simulink library "rocket_isa_model_library"  (R2014a)
settings: Solver=ode45  StartTime=0.0  StopTime=10.0  RelTol=1e-3
settings Model: Creator=scorpii  LastModifiedBy=scorpii

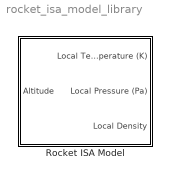
== system rocket_isa_model_library ==
  Rocket ISA Model : Subsystem

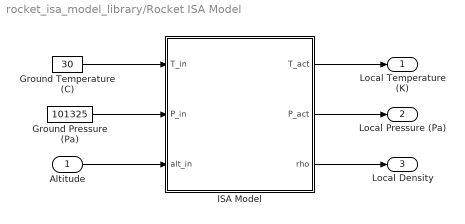
== system rocket_isa_model_library/Rocket ISA Model ==
  Altitude : Inport
  Ground Pressure (Pa) : Constant  Value=101325
  Ground Temperature (C) : Constant  Value=30
  ISA Model : Subsystem
  Local Temperature (K) : Outport
  Local Pressure (Pa) : Outport  Port=2
  Local Density : Outport  Port=3
  wires:
  Ground Temperature (C)/1 -> ISA Model/1(T_in)
  Ground Pressure (Pa)/1 -> ISA Model/2(P_in)
  Altitude/1 -> ISA Model/3(alt_in)
  ISA Model/1(T_act) -> Local Temperature (K)/1
  ISA Model/2(P_act) -> Local Pressure (Pa)/1
  ISA Model/3(rho) -> Local Density/1

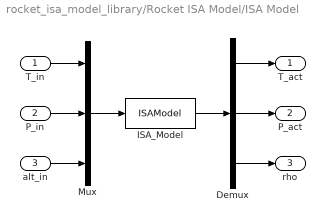
== system rocket_isa_model_library/Rocket ISA Model/ISA Model ==
  T_in : Inport
  P_in : Inport  Port=2
  alt_in : Inport  Port=3
  Demux : Demux  Outputs=3
  ISA_Model : MATLABFcn  MATLABFcn=ISAModel
      mask Display: disp('ISAModel')
  Mux : Mux  Inputs=3
  T_act : Outport
  P_act : Outport  Port=2
  rho : Outport  Port=3
  wires:
  alt_in/1 -> Mux/3
  P_in/1 -> Mux/2
  Demux/2 -> P_act/1
  Mux/1 -> ISA_Model/1
  T_in/1 -> Mux/1
  Demux/1 -> T_act/1
  Demux/3 -> rho/1
  ISA_Model/1 -> Demux/1
